simulink model "LE1"  (R2021a)
settings: Solver=FixedStepDiscrete  StartTime=0.0  StopTime=4  RelTol=1e-3
libraries: dsparch4 x1
settings Model: Creator=antho  LastModifiedBy=antho

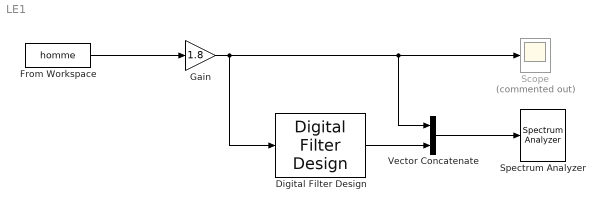
== system LE1 ==
  Digital Filter Design : dsparch4/Digital Filter Design  mwdsp_browser_bugfix_var=off
  From Workspace : FromWorkspace  VariableName=homme  SampleTime=1/16000
  Gain : Gain  Gain=1.8
  Scope : Scope  Commented=on
  Spectrum Analyzer : SpectrumAnalyzer
  Vector Concatenate : Concatenate  Mode=Multidimensional array  ConcatenateDimension=2
  wires:
  From Workspace/1 -> Gain/1
  Gain/1 -> Digital Filter Design/1, Vector Concatenate/1, Scope/1
  Digital Filter Design/1 -> Vector Concatenate/2
  Vector Concatenate/1 -> Spectrum Analyzer/1
